simulink model "LMS_FILTER_4_TAP"  (R2016a)
settings: Solver=VariableStepDiscrete  StartTime=0.0  StopTime=3000  MaxStep=1.0  RelTol=1e-3
libraries: dspsrcs4 x2, dspstat3 x2, dspmathops x1
settings Model: Creator=HP  LastModifiedBy=HP

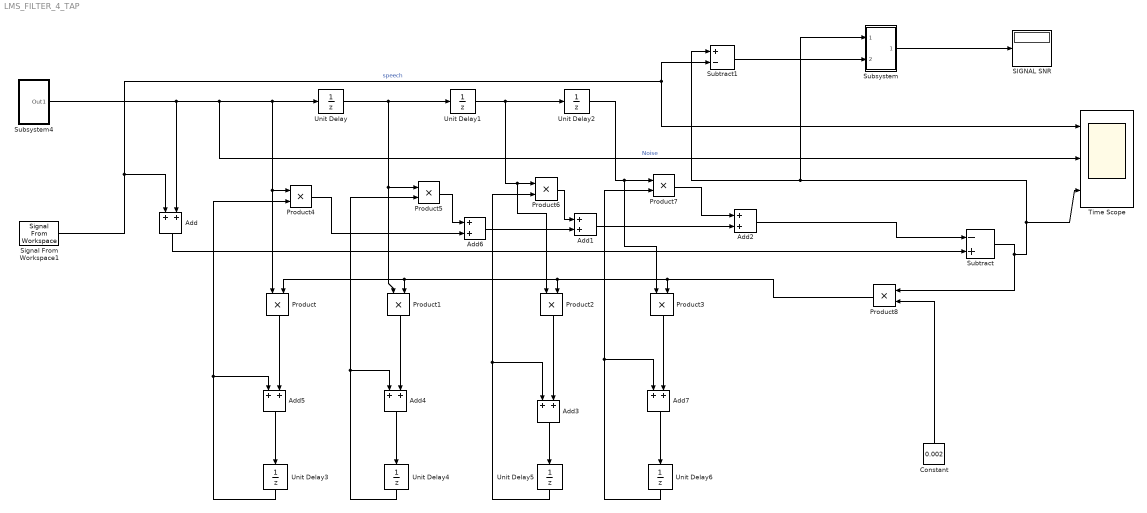
== system LMS_FILTER_4_TAP ==
  Add{,1..7} (8 alike) : Sum
  Constant : Constant  Value=0.002
  Product{,1..8} (9 alike) : Product
  "SIGNAL SNR " : Display
  Signal From Workspace1 : dspsrcs4/Signal From Workspace  X=m1  Ts=1  nsamps=1  OutputAfterFinalValue=Setting to zero  ignoreOrWarnInputAndFrameLengths=off  OutputFrames=off
  Subsystem : Subsystem
  Subsystem4 : Subsystem
  Subtract : Sum  Inputs=-+
  Subtract1 : Sum  Inputs=+-
  Time Scope : Scope  NumInputPorts=3
  Unit Delay{,1..6} (7 alike) : UnitDelay  SampleTime=-1
  wires:
  Unit Delay/1 -> Product5/1, Product1/1, Unit Delay1/1
  Unit Delay1/1 -> Product2/1, Product6/1, Unit Delay2/1
  Unit Delay2/1 -> Product7/1, Product3/1
  Signal From Workspace1/1 -> Time Scope/1, Subtract1/2, Add/1  "speech"
  Unit Delay3/1 -> Add5/1, Product4/2
  Product/1 -> Add5/2
  Product8/1 -> Product/2, Product1/2, Product2/2, Product3/2
  Unit Delay4/1 -> Add4/1, Product5/2
  Add5/1 -> Unit Delay3/1
  Add4/1 -> Unit Delay4/1
  Product1/1 -> Add4/2
  Product5/1 -> Add6/1
  Product4/1 -> Add6/2
  Product2/1 -> Add3/2
  Unit Delay5/1 -> Add3/1, Product6/2
  Add3/1 -> Unit Delay5/1
  Product6/1 -> Add1/1
  Add6/1 -> Add1/2
  Unit Delay6/1 -> Add7/1, Product7/2
  Product3/1 -> Add7/2
  Product7/1 -> Add2/1
  Add1/1 -> Add2/2
  Add7/1 -> Unit Delay6/1
  Constant/1 -> Product8/2
  Add/1 -> Subtract/2
  Add2/1 -> Subtract/1
  Subtract1/1 -> Subsystem/2(In2)
  Subsystem/1(Out1) -> "SIGNAL SNR "/1
  Subsystem4/1(Out1) -> Time Scope/2, Product4/1, Product/1, Unit Delay/1, Add/2  "Noise"
  Subtract/1 -> Product8/1, Subsystem/1(In1), Subtract1/1, Time Scope/3

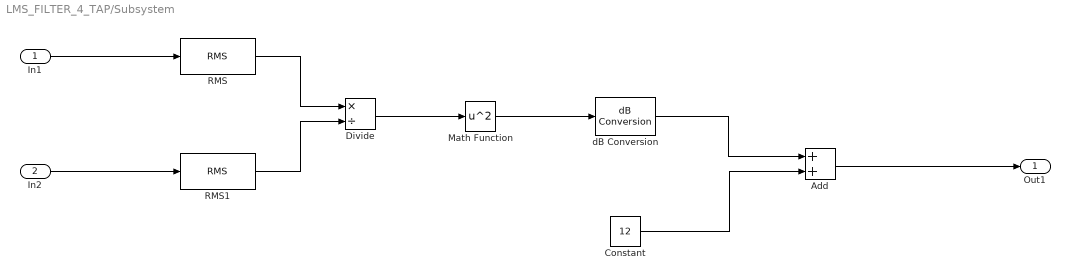
== system LMS_FILTER_4_TAP/Subsystem ==
  In1 : Inport
  In2 : Inport  Port=2
  Add : Sum
  Constant : Constant  Value=12
  Divide : Product  Inputs=*/
  Math Function : Math  Operator=square  OutputSignalType=real  SaturateOnIntegerOverflow=on
  RMS : dspstat3/RMS  run=on  reset_popup=None  InputProcessing=Columns as channels (frame based)  directionMode=Each column  dimension=1
  RMS1 : dspstat3/RMS  run=on  reset_popup=None  InputProcessing=Columns as channels (frame based)  directionMode=Each column  dimension=1
  dB Conversion : dspmathops/dB Conversion  dBtype=dB  intype=Amplitude  R=1  fuzz=off
  Out1 : Outport
  wires:
  RMS1/1 -> Divide/2
  dB Conversion/1 -> Add/1
  In1/1 -> RMS/1
  Divide/1 -> Math Function/1
  RMS/1 -> Divide/1
  In2/1 -> RMS1/1
  Add/1 -> Out1/1
  Constant/1 -> Add/2
  Math Function/1 -> dB Conversion/1

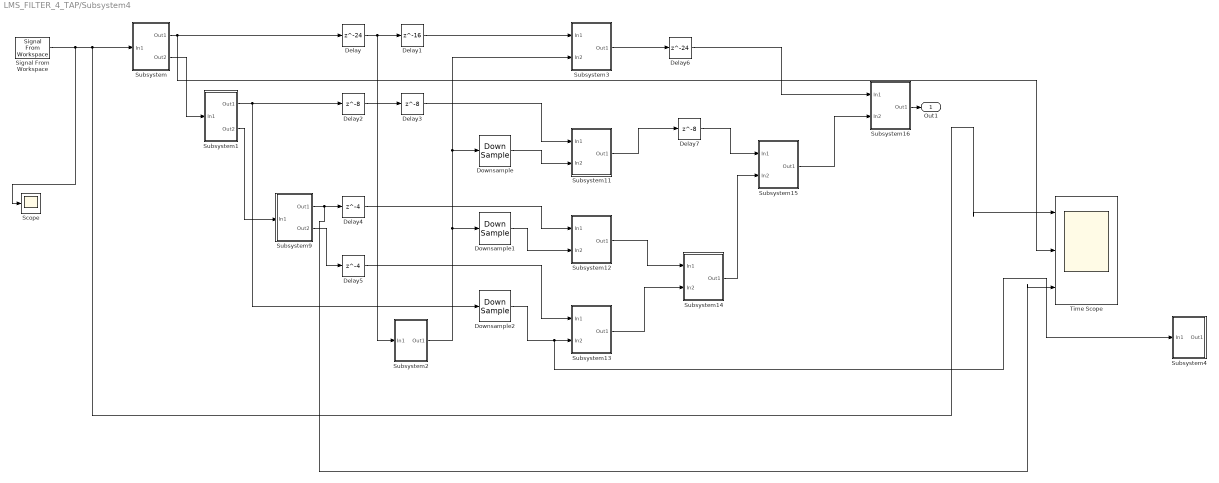
== system LMS_FILTER_4_TAP/Subsystem4 ==
  Delay : Delay  DelayLength=24  InitialCondition=0
  Delay1 : Delay  DelayLength=16  InitialCondition=0
  Delay2 : Delay  DelayLength=8  InitialCondition=0
  Delay3 : Delay  DelayLength=8  InitialCondition=0
  Delay4 : Delay  DelayLength=4  InitialCondition=0
  Delay5 : Delay  DelayLength=4  InitialCondition=0
  Delay6 : Delay  DelayLength=24  InitialCondition=0
  Delay7 : Delay  DelayLength=8  InitialCondition=0
  Downsample : DownSample  RateOptions=Allow multirate processing  ic=-1
  Downsample1 : DownSample  N=4  RateOptions=Allow multirate processing  ic=-1
  Downsample2 : DownSample  N=8  phase=1  ic=-1
  Scope : Scope
  Signal From Workspace : dspsrcs4/Signal From Workspace  X=y  Ts=1  nsamps=1  OutputAfterFinalValue=Setting to zero  ignoreOrWarnInputAndFrameLengths=off  OutputFrames=off
  Subsystem : Subsystem
  Subsystem1 : Subsystem
  Subsystem11 : Subsystem
  Subsystem12 : Subsystem
  Subsystem13 : Subsystem
  Subsystem14 : Subsystem
  Subsystem15 : Subsystem
  Subsystem16 : Subsystem
  Subsystem2 : Subsystem
  Subsystem3 : Subsystem
  Subsystem4 : Subsystem
  Subsystem9 : Subsystem
  Time Scope : Scope  NumInputPorts=3
  Out1 : Outport
  wires:
  Subsystem1/2(Out2) -> Subsystem9/1(In1)
  Delay3/1 -> Subsystem11/1(In1)
  Downsample/1 -> Subsystem11/2(In2)
  Subsystem9/1(Out1) -> Time Scope/3, Delay4/1
  Subsystem/1(Out1) -> Time Scope/2, Delay/1
  Signal From Workspace/1 -> Scope/1, Time Scope/1, Subsystem/1(In1)
  Subsystem/2(Out2) -> Subsystem1/1(In1)
  Delay2/1 -> Delay3/1
  Subsystem11/1(Out1) -> Delay7/1
  Delay1/1 -> Subsystem3/1(In1)
  Delay/1 -> Subsystem2/1(In1), Delay1/1
  Delay4/1 -> Subsystem12/1(In1)
  Downsample2/1 -> Subsystem4/1(In1), Subsystem13/2(In2)
  Subsystem13/1(Out1) -> Subsystem14/2(In2)
  Subsystem3/1(Out1) -> Delay6/1
  Delay6/1 -> Subsystem16/1(In1)
  Subsystem1/1(Out1) -> Delay2/1, Downsample2/1
  Subsystem15/1(Out1) -> Subsystem16/2(In2)
  Subsystem14/1(Out1) -> Subsystem15/2(In2)
  Subsystem9/2(Out2) -> Delay5/1
  Downsample1/1 -> Subsystem12/2(In2)
  Delay5/1 -> Subsystem13/1(In1)
  Subsystem12/1(Out1) -> Subsystem14/1(In1)
  Delay7/1 -> Subsystem15/1(In1)
  Subsystem2/1(Out1) -> Downsample1/1, Subsystem3/2(In2), Downsample/1
  Subsystem16/1(Out1) -> Out1/1

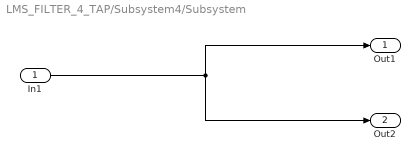
== system LMS_FILTER_4_TAP/Subsystem4/Subsystem ==
  In1 : Inport
  Out1 : Outport
  Out2 : Outport  Port=2
  wires:
  In1/1 -> Out1/1, Out2/1

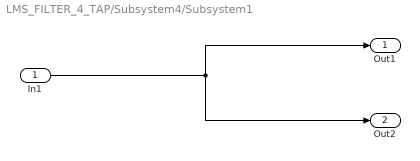
== system LMS_FILTER_4_TAP/Subsystem4/Subsystem1 ==
  In1 : Inport
  Out1 : Outport
  Out2 : Outport  Port=2
  wires:
  In1/1 -> Out1/1, Out2/1

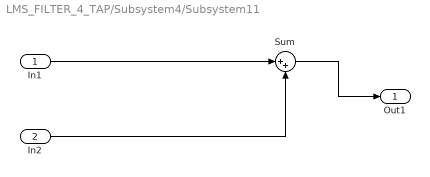
== system LMS_FILTER_4_TAP/Subsystem4/Subsystem11 ==
  In1 : Inport
  In2 : Inport  Port=2
  Sum : Sum  Inputs=|++
  Out1 : Outport
  wires:
  In1/1 -> Sum/1
  In2/1 -> Sum/2
  Sum/1 -> Out1/1

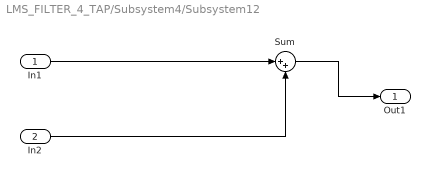
== system LMS_FILTER_4_TAP/Subsystem4/Subsystem12 ==
  In1 : Inport
  In2 : Inport  Port=2
  Sum : Sum  Inputs=|++
  Out1 : Outport
  wires:
  In1/1 -> Sum/1
  In2/1 -> Sum/2
  Sum/1 -> Out1/1

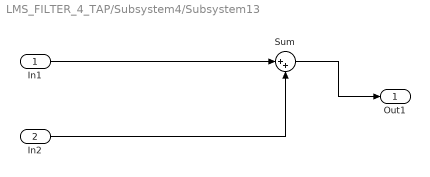
== system LMS_FILTER_4_TAP/Subsystem4/Subsystem13 ==
  In1 : Inport
  In2 : Inport  Port=2
  Sum : Sum  Inputs=|++
  Out1 : Outport
  wires:
  In1/1 -> Sum/1
  In2/1 -> Sum/2
  Sum/1 -> Out1/1

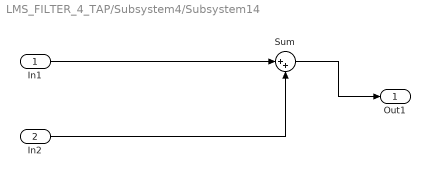
== system LMS_FILTER_4_TAP/Subsystem4/Subsystem14 ==
  In1 : Inport
  In2 : Inport  Port=2
  Sum : Sum  Inputs=|++
  Out1 : Outport
  wires:
  In1/1 -> Sum/1
  In2/1 -> Sum/2
  Sum/1 -> Out1/1

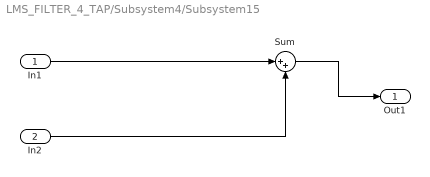
== system LMS_FILTER_4_TAP/Subsystem4/Subsystem15 ==
  In1 : Inport
  In2 : Inport  Port=2
  Sum : Sum  Inputs=|++
  Out1 : Outport
  wires:
  In1/1 -> Sum/1
  In2/1 -> Sum/2
  Sum/1 -> Out1/1

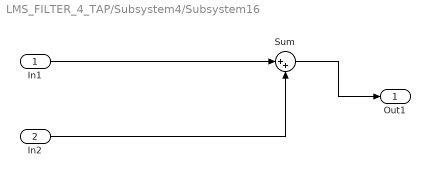
== system LMS_FILTER_4_TAP/Subsystem4/Subsystem16 ==
  In1 : Inport
  In2 : Inport  Port=2
  Sum : Sum  Inputs=|++
  Out1 : Outport
  wires:
  In1/1 -> Sum/1
  In2/1 -> Sum/2
  Sum/1 -> Out1/1

== system LMS_FILTER_4_TAP/Subsystem4/Subsystem2 ==
  In1 : Inport
  Out1 : Outport
  wires:
  In1/1 -> Out1/1

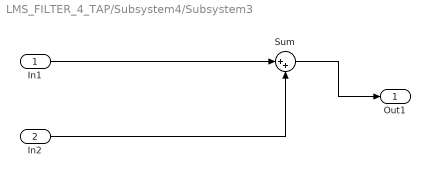
== system LMS_FILTER_4_TAP/Subsystem4/Subsystem3 ==
  In1 : Inport
  In2 : Inport  Port=2
  Sum : Sum  Inputs=|++
  Out1 : Outport
  wires:
  In1/1 -> Sum/1
  In2/1 -> Sum/2
  Sum/1 -> Out1/1

== system LMS_FILTER_4_TAP/Subsystem4/Subsystem4 ==
  In1 : Inport
  Out1 : Outport
  wires:
  In1/1 -> Out1/1

== system LMS_FILTER_4_TAP/Subsystem4/Subsystem9 ==
  In1 : Inport
  Out1 : Outport
  Out2 : Outport  Port=2
  wires:
  In1/1 -> Out1/1, Out2/1
